simulink library "CTRL_SPECCTRL_FB_STRAT1_YAWM"  (R2024b)
settings: Solver=VariableStepAuto  StartTime=0.0  StopTime=10.0  RelTol=1e-3
undefined symbols (not defined in the file): p_trackFr_m, p_trackRe_m
settings Model: Creator=blatak  LastModifiedBy=blatak

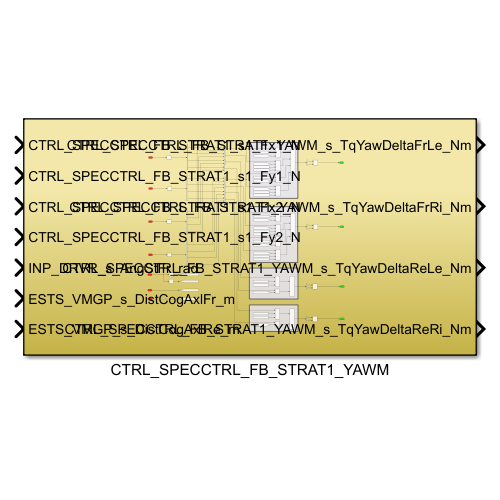
[thumbnail: Simulink's stored preview of the top-level diagram]
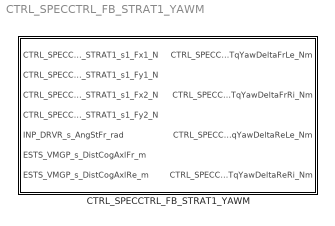
== system CTRL_SPECCTRL_FB_STRAT1_YAWM ==
  CTRL_SPECCTRL_FB_STRAT1_YAWM : Subsystem

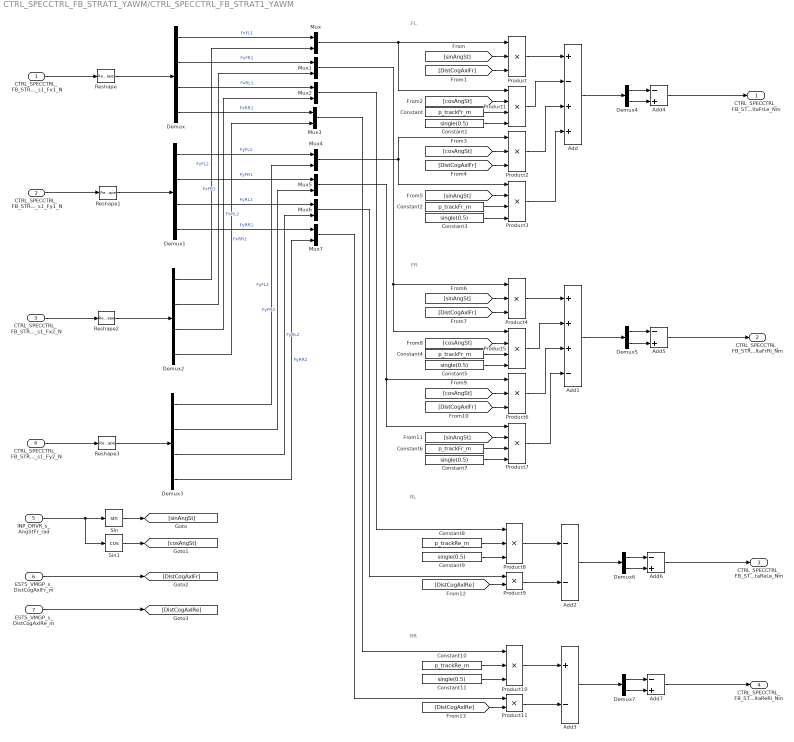
== system CTRL_SPECCTRL_FB_STRAT1_YAWM/CTRL_SPECCTRL_FB_STRAT1_YAWM ==
  note: RR
  note: RL
  note: FR
  note: FL
  CTRL_SPECCTRL_FB_STRAT1_s1_Fx1_N : Inport
  CTRL_SPECCTRL_FB_STRAT1_s1_Fy1_N : Inport  Port=2
  CTRL_SPECCTRL_FB_STRAT1_s1_Fx2_N : Inport  Port=3
  CTRL_SPECCTRL_FB_STRAT1_s1_Fy2_N : Inport  Port=4
  INP_DRVR_s_AngStFr_rad : Inport  Port=5
  ESTS_VMGP_s_DistCogAxlFr_m : Inport  Port=6
  ESTS_VMGP_s_DistCogAxlRe_m : Inport  Port=7
  Add : Sum  Inputs=+-++
  Add1 : Sum  Inputs=+++-
  Add2 : Sum  Inputs=--
  Add3 : Sum  Inputs=+-
  Add{4..7} (4 alike) : Sum  Inputs=-+
  Constant{,2,4,6} (4 alike) : Constant  Value=p_trackFr_m
  Constant{1,3,5,7,9,11} (6 alike) : Constant  Value=single(0.5)
  Constant10 : Constant  Value=p_trackRe_m
  Constant8 : Constant  Value=p_trackRe_m
  Demux{,1..3} (4 alike) : Demux
  Demux{4..7} (4 alike) : Demux  Outputs=2
  Mux{,1..7} (8 alike) : Mux  Inputs=2
  Product{,2,4,6,8,10} (6 alike) : Product  Inputs=3
  Product{1,3,5,7} (4 alike) : Product  Inputs=4
  Product11 : Product
  Product9 : Product
  Reshape{,1..3} (4 alike) : Reshape
  Sin : Trigonometry
  Sin1 : Trigonometry  Operator=cos
  CTRL_SPECCTRL_FB_STRAT1_YAWM_s_TqYawDeltaFrLe_Nm : Outport
  CTRL_SPECCTRL_FB_STRAT1_YAWM_s_TqYawDeltaFrRi_Nm : Outport  Port=2
  CTRL_SPECCTRL_FB_STRAT1_YAWM_s_TqYawDeltaReLe_Nm : Outport  Port=3
  CTRL_SPECCTRL_FB_STRAT1_YAWM_s_TqYawDeltaReRi_Nm : Outport  Port=4
  wires:
  CTRL_SPECCTRL_FB_STRAT1_s1_Fx1_N/1 -> Reshape/1
  Reshape/1 -> Demux/1
  CTRL_SPECCTRL_FB_STRAT1_s1_Fy1_N/1 -> Reshape1/1
  Reshape1/1 -> Demux1/1
  CTRL_SPECCTRL_FB_STRAT1_s1_Fx2_N/1 -> Reshape2/1
  Reshape2/1 -> Demux2/1
  CTRL_SPECCTRL_FB_STRAT1_s1_Fy2_N/1 -> Reshape3/1
  Reshape3/1 -> Demux3/1
  Demux/1 -> Mux/1  "FxFL1"
  Demux2/1 -> Mux/2  "FxFL2"
  Demux/2 -> Mux1/1  "FxFR1"
  Demux2/2 -> Mux1/2  "FxFR2"
  Demux/3 -> Mux2/1  "FxRL1"
  Demux2/3 -> Mux2/2  "FxRL2"
  Demux/4 -> Mux3/1  "FxRR1"
  Demux2/4 -> Mux3/2  "FxRR2"
  Demux1/2 -> Mux5/1  "FyFR1"
  Demux1/3 -> Mux6/1  "FyRL1"
  Demux3/3 -> Mux6/2  "FyRL2"
  Demux3/2 -> Mux5/2  "FyFR2"
  Demux3/1 -> Mux4/2  "FyFL2"
  Demux3/4 -> Mux7/2  "FyRR2"
  Demux1/1 -> Mux4/1  "FyFL1"
  Demux1/4 -> Mux7/1  "FyRR1"
  INP_DRVR_s_AngStFr_rad/1 -> Sin1/1, Sin/1
  Sin/1 -> [sinAngSt]
  Sin1/1 -> [cosAngSt]
  ESTS_VMGP_s_DistCogAxlFr_m/1 -> [DistCogAxlFr]
  ESTS_VMGP_s_DistCogAxlRe_m/1 -> [DistCogAxlRe]
  Add/1 -> Demux4/1
  Product3/1 -> Add/4
  Product/1 -> Add/1
  [cosAngSt] -> Product1/2
  [sinAngSt] -> Product/2
  [DistCogAxlFr] -> Product2/3
  [sinAngSt] -> Product3/2
  Mux/1 -> Product1/1, Product/1
  [cosAngSt] -> Product2/2
  Product2/1 -> Add/3
  Constant/1 -> Product1/3
  Constant1/1 -> Product1/4
  Constant3/1 -> Product3/4
  [DistCogAxlFr] -> Product/3
  Mux4/1 -> Product3/1, Product2/1
  Product1/1 -> Add/2
  Constant2/1 -> Product3/3
  Constant6/1 -> Product7/3
  Mux1/1 -> Product5/1, Product4/1
  Product6/1 -> Add1/3
  [DistCogAxlFr] -> Product4/3
  [cosAngSt] -> Product5/2
  [DistCogAxlFr] -> Product6/3
  [sinAngSt] -> Product7/2
  [sinAngSt] -> Product4/2
  [cosAngSt] -> Product6/2
  Constant4/1 -> Product5/3
  Constant5/1 -> Product5/4
  Product4/1 -> Add1/1
  Constant7/1 -> Product7/4
  Mux5/1 -> Product7/1, Product6/1
  Product5/1 -> Add1/2
  Product7/1 -> Add1/4
  Product9/1 -> Add2/2
  Constant8/1 -> Product8/2
  Constant9/1 -> Product8/3
  Product8/1 -> Add2/1
  Mux2/1 -> Product8/1
  Mux6/1 -> Product9/1
  [DistCogAxlRe] -> Product9/2
  Mux3/1 -> Product10/1
  Mux7/1 -> Product11/1
  Product11/1 -> Add3/2
  [DistCogAxlRe] -> Product11/2
  Product10/1 -> Add3/1
  Constant10/1 -> Product10/2
  Constant11/1 -> Product10/3
  Demux4/1 -> Add4/1
  Demux4/2 -> Add4/2
  Demux5/1 -> Add5/1
  Add1/1 -> Demux5/1
  Demux5/2 -> Add5/2
  Demux6/1 -> Add6/1
  Add2/1 -> Demux6/1
  Demux6/2 -> Add6/2
  Demux7/1 -> Add7/1
  Add3/1 -> Demux7/1
  Demux7/2 -> Add7/2
  Add4/1 -> CTRL_SPECCTRL_FB_STRAT1_YAWM_s_TqYawDeltaFrLe_Nm/1
  Add5/1 -> CTRL_SPECCTRL_FB_STRAT1_YAWM_s_TqYawDeltaFrRi_Nm/1
  Add6/1 -> CTRL_SPECCTRL_FB_STRAT1_YAWM_s_TqYawDeltaReLe_Nm/1
  Add7/1 -> CTRL_SPECCTRL_FB_STRAT1_YAWM_s_TqYawDeltaReRi_Nm/1
